simulink model "EnabledSubsystem_modelA"  (R2018b)
settings: Solver=FixedStepAuto  StartTime=0.0  StopTime=tFinal  FixedStep=deltaT  RelTol=1e-3
values from neighbouring files (symbols this model uses):
  x0 = 50    [MAIN_EnabledSubsystem.m]
libraries: simulink x1
settings Model: Creator=Christopher  LastModifiedBy=Christopher

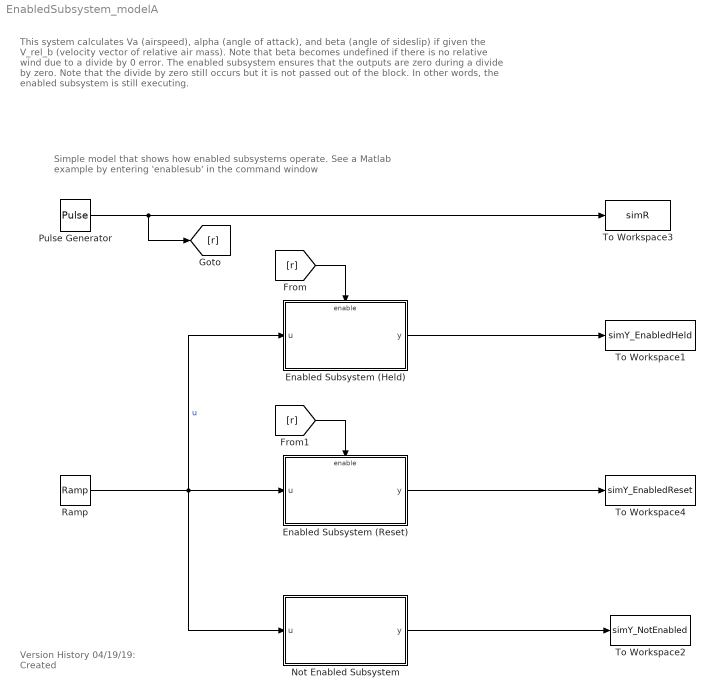
== system EnabledSubsystem_modelA ==
  note: Simple model that shows how enabled subsystems operate.
      |
      | See a Matlab example by entering 'enablesub' in the command window
  note: This system calculates Va (airspeed), alpha (angle of attack), and beta (angle of sideslip) if given the V_rel_b (velocity vector of relative air mass).
      |
      | Note that beta becomes undefined if there is no relative wind due to a divide by 0 error.
      |
      | The enabled subsystem ensures that the outputs are zero during a divide by zero.  Note that the divide by zero still occurs but it is not passed out of the block.  In other words, the enabled subsystem is still executing.
  note: Version History
      | 04/19/19: Created
  Enabled Subsystem (Held) : Subsystem
  Enabled Subsystem (Reset) : Subsystem
  Not Enabled Subsystem : Subsystem
  Pulse Generator : DiscretePulseGenerator  PulseType=Time based  Period=8  PulseWidth=75
  Ramp : simulink/Sources/Ramp  slope=1  start=0  InitialOutput=0
  To Workspace1 : ToWorkspace  VariableName=simY_EnabledHeld  SaveFormat=Timeseries  SampleTime=-1
  To Workspace2 : ToWorkspace  VariableName=simY_NotEnabled  SaveFormat=Timeseries  SampleTime=-1
  To Workspace3 : ToWorkspace  VariableName=simR  SaveFormat=Timeseries  SampleTime=-1
  To Workspace4 : ToWorkspace  VariableName=simY_EnabledReset  SaveFormat=Timeseries  SampleTime=-1
  wires:
  Ramp/1 -> Not Enabled Subsystem/1(u), Enabled Subsystem (Held)/1(u), Enabled Subsystem (Reset)/1(u)  "u"
  Enabled Subsystem (Held)/1(y) -> To Workspace1/1
  Pulse Generator/1 -> [r], To Workspace3/1
  [r] -> Enabled Subsystem (Held)/Enable
  [r] -> Enabled Subsystem (Reset)/Enable
  Enabled Subsystem (Reset)/1(y) -> To Workspace4/1
  Not Enabled Subsystem/1(y) -> To Workspace2/1

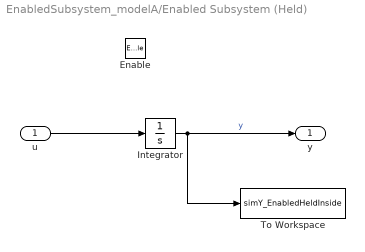
== system EnabledSubsystem_modelA/Enabled Subsystem (Held) ==
  u : Inport
  Enable : EnablePort
  Integrator : Integrator  InitialCondition=x0
  To Workspace : ToWorkspace  VariableName=simY_EnabledHeldInside  SaveFormat=Timeseries  SampleTime=-1
  y : Outport
  wires:
  u/1 -> Integrator/1
  Integrator/1 -> To Workspace/1, y/1  "y"

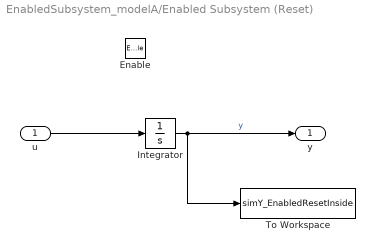
== system EnabledSubsystem_modelA/Enabled Subsystem (Reset) ==
  u : Inport
  Enable : EnablePort  StatesWhenEnabling=reset
  Integrator : Integrator  InitialCondition=x0
  To Workspace : ToWorkspace  VariableName=simY_EnabledResetInside  SaveFormat=Timeseries  SampleTime=-1
  y : Outport
  wires:
  Integrator/1 -> y/1, To Workspace/1  "y"
  u/1 -> Integrator/1

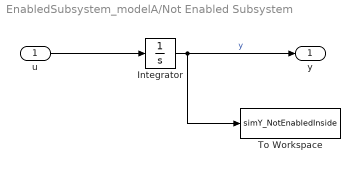
== system EnabledSubsystem_modelA/Not Enabled Subsystem ==
  u : Inport
  Integrator : Integrator  InitialCondition=x0
  To Workspace : ToWorkspace  VariableName=simY_NotEnabledInside  SaveFormat=Timeseries  SampleTime=-1
  y : Outport
  wires:
  u/1 -> Integrator/1
  Integrator/1 -> To Workspace/1, y/1  "y"
